simulink model "my_foc_TI"  (R2021b)
settings: Solver=ode23t  StartTime=0.0  StopTime=1  FixedStep=0.0000001  RelTol=1e-7  EnableMultiTasking=on
InitFcn:
  | Ld=5.25e-3;
  | Lq=12e-3;
  | R=0.958;
  | f=0.1827;
model workspace (MAT data in the model file):
  f = Simulink.Signal
  f.DataType = 'single'
  f.Dimensions = 1
  f.DimensionsMode = 'auto'
  f.Complexity = 'real'
  f.SampleTime = -1
  f.SamplingMode = 'auto'
  f.InitialValue = '0.1827'
undefined symbols (not defined in the file or in its folder): sigbuilder_block
libraries: slpidlib x7, simulink x3, SignalEditorBlockLib x2, mcbplantlib x1, spsPermanentMagnetSynchronousMachineLib x1, autolibpmsmexterior x1, spspowerguiLib x1
settings Model: Creator=张豪  LastModifiedBy=LingweiWRB
settings SolverCC: AutoInsertRateTranBlk=on

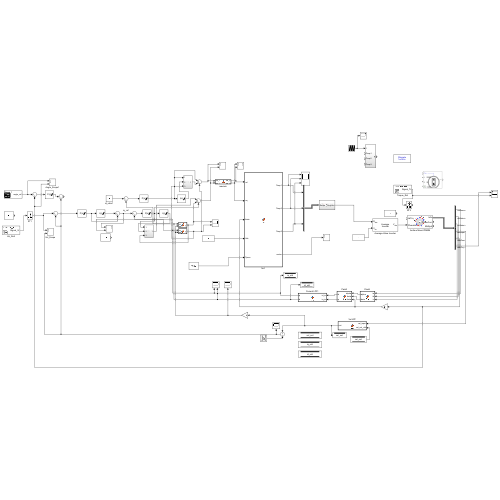
[thumbnail: Simulink's stored preview of the top-level diagram]
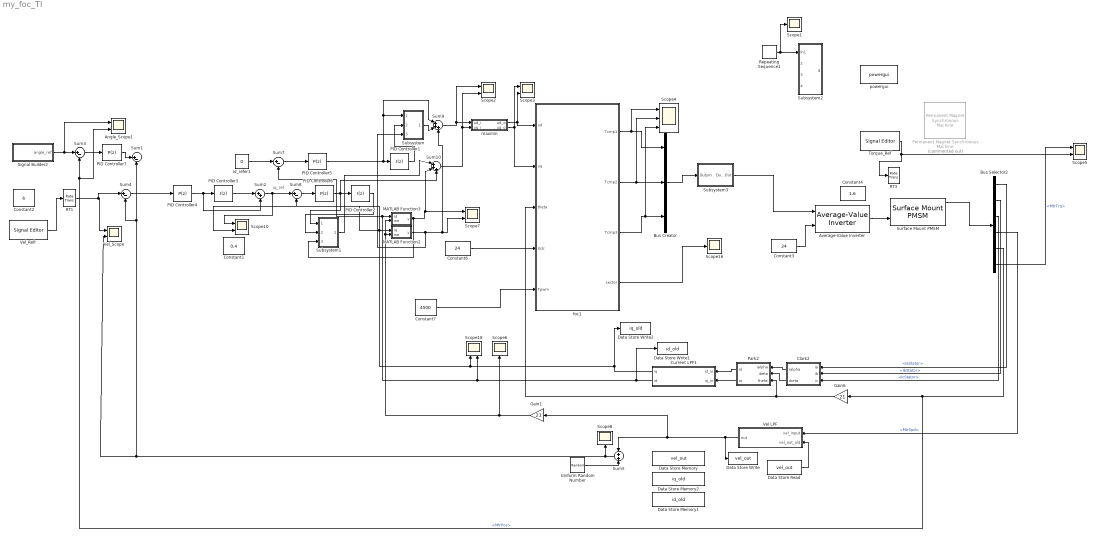
== system my_foc_TI ==
  note: iq_ref
  Angle_Scope1 : Scope  NumInputPorts=2
  Average-Value Inverter : mcbplantlib/Average-Value Inverter
  Bus Creator : BusCreator  Inputs=3
  Bus Selector2 : BusSelector  OutputSignals=IaStator,IbStator,IcStator,MtrSpd,MtrPos,MtrTrq
  Clark2 : MATLAB Function  TreatAsAtomicUnit=on
  Constant1 : Constant  Value=0.4  OutDataTypeStr=single
  Constant2 : Constant  Value=6  OutDataTypeStr=single
  Constant3 : Constant  Value=24
  Constant4 : Constant  Value=1.6
  Constant6 : Constant  Value=24
  Constant7 : Constant  Value=4500  OutDataTypeStr=single
  Current LPF1 : MATLAB Function  TreatAsAtomicUnit=on
  Data Store Memory : DataStoreMemory  DataStoreName=vel_out  ReadBeforeWriteMsg=warning  WriteAfterWriteMsg=warning  WriteAfterReadMsg=warning  ShowAdditionalParam=off  OutDataTypeStr=double
  Data Store Memory1 : DataStoreMemory  DataStoreName=id_old  ReadBeforeWriteMsg=warning  WriteAfterWriteMsg=warning  WriteAfterReadMsg=warning  ShowAdditionalParam=off  OutDataTypeStr=double
  Data Store Memory2 : DataStoreMemory  DataStoreName=iq_old  ReadBeforeWriteMsg=warning  WriteAfterWriteMsg=warning  WriteAfterReadMsg=warning  ShowAdditionalParam=off  OutDataTypeStr=double
  Data Store Read : DataStoreRead  DataStoreName=vel_out  DataStoreElements=vel_out  IndexOptions=Index vector (dialog)  Indices=1  OutputSizes=1
  Data Store Write : DataStoreWrite  DataStoreName=vel_out  DataStoreElements=vel_out  IndexOptions=Index vector (dialog)  Indices=1  OutputSizes=1
  Data Store Write1 : DataStoreWrite  DataStoreName=id_old  DataStoreElements=id_old  IndexOptions=Index vector (dialog)  Indices=1  OutputSizes=1
  Data Store Write2 : DataStoreWrite  DataStoreName=iq_old  DataStoreElements=iq_old  IndexOptions=Index vector (dialog)  Indices=1  OutputSizes=1
  Gain1 : Gain  Gain=21
  Gain6 : Gain  Gain=21
  MATLAB Function2 : MATLAB Function  TreatAsAtomicUnit=on
  MATLAB Function3 : MATLAB Function  TreatAsAtomicUnit=on
  PID Controller1 : slpidlib/PID Controller  Controller=I  Form=Parallel  TimeDomain=Discrete-time  UseExternalTs=off  SampleTime=-1  IntegratorMethod=Forward Euler  FilterMethod=Forward Euler  ControllerParametersSource=internal  P=3.768  I=406.4740  D=0  UseFilter=on  N=100  TunerSelectOption=Transfer Function Based (PID Tuner App)  InitialConditionSource=internal  InitialConditionForIntegrator=0  InitialConditionForFilter=0  DifferentiatorICPrevScaledInput=0  ExternalReset=none  TrackingMode=off  Kt=1  LimitOutput=on  SatLimitsSource=internal  UpperSaturationLimit=36  LowerSaturationLimit=-36  LinearizeAsGain=on  AntiWindupMode=none  Kb=1  POutMin=[]  POutMax=[]  IOutMin=[]  IOutMax=[]  DOutMin=[]  DOutMax=[]  NOutMin=[]  NOutMax=[]  SumOutMin=[]  SumOutMax=[]  SaturationOutMin=[]  SaturationOutMax=[]  PParamMin=[]  PParamMax=[]  IParamMin=[]  IParamMax=[]  DParamMin=[]  DParamMax=[]  NParamMin=[]  NParamMax=[]  KbParamMin=[]  KbParamMax=[]  KtParamMin=[]  KtParamMax=[]  KbOutMin=[]  KbOutMax=[]  KtOutMin=[]  KtOutMax=[]  IntegratorOutMin=[]  IntegratorOutMax=[]  FilterOutMin=[]  FilterOutMax=[]  SumI1OutMin=[]  SumI1OutMax=[]  SumI2OutMin=[]  SumI2OutMax=[]  SumI3OutMin=[]  SumI3OutMax=[]  SumI4OutMin=[]  SumI4OutMax=[]  SumDOutMin=[]  SumDOutMax=[]  DifferentiatorOutMin=[]  DifferentiatorOutMax=[]  FilterDiffOutCoefMin=[]  FilterDiffOutCoefMax=[]  ReciprocalOutMin=[]  ReciprocalOutMax=[]  SumDenOutMin=[]  SumDenOutMax=[]  SumNumOutMin=[]  SumNumOutMax=[]  DivideOutMin=[]  DivideOutMax=[]  UdiffTsProdOutMin=[]  UdiffTsProdOutMax=[]  NTsProdOutMin=[]  NTsProdOutMax=[]  UintegralTsProdOutMin=[]  UintegralTsProdOutMax=[]  UngainTsProdOutMin=[]  UngainTsProdOutMax=[]  IntegratorContinuousStateAttributes=''  IntegratorStateMustResolveToSignalObject=off  IntegratorRTWStateStorageClass=Auto  FilterContinuousStateAttributes=''  FilterStateMustResolveToSignalObject=off  FilterRTWStateStorageClass=Auto  ParallelPVariant=Disabled  IdealPVariant=Disabled  IVariant=InternalParameters  DVariant=Disabled  IntegratorVariant=Discrete  SatVariant=Enabled  AWVariant=Passthrough  PCopyVariant=Disabled  TRVariant=Disabled  FdbkBlocksVariant=Forward  IdealPFdbkVariant=Disabled  SatFdbkVariant=Disabled  DerivativeFilterVariant=Disabled  NVariant=Disabled  NCopyVariant=Disabled_SignalSpec  FilterICVariant=Disabled  IntegratorICVariant=InternalICs  ExternalResetVariant=Disabled  TRSumVariant=Passthrough  SumFdbkVariant=Disabled  SumVariant=Passthrough_I  TsampFilterVariant=InternalTs  TsampNgainVariant=Passthrough  TsampIntegralVariant=Passthrough  ExternalSaturationOutDataTypeStr=Inherit: Same as second input
  PID Controller2 : slpidlib/PID Controller  Controller=I  Form=Parallel  TimeDomain=Discrete-time  UseExternalTs=off  SampleTime=-1  IntegratorMethod=Forward Euler  FilterMethod=Forward Euler  ControllerParametersSource=internal  P=3.768  I=406.4740  D=0  UseFilter=on  N=100  TunerSelectOption=Transfer Function Based (PID Tuner App)  InitialConditionSource=internal  InitialConditionForIntegrator=0  InitialConditionForFilter=0  DifferentiatorICPrevScaledInput=0  ExternalReset=none  TrackingMode=off  Kt=1  LimitOutput=on  SatLimitsSource=internal  UpperSaturationLimit=36  LowerSaturationLimit=-36  LinearizeAsGain=on  AntiWindupMode=none  Kb=1  POutMin=[]  POutMax=[]  IOutMin=[]  IOutMax=[]  DOutMin=[]  DOutMax=[]  NOutMin=[]  NOutMax=[]  SumOutMin=[]  SumOutMax=[]  SaturationOutMin=[]  SaturationOutMax=[]  PParamMin=[]  PParamMax=[]  IParamMin=[]  IParamMax=[]  DParamMin=[]  DParamMax=[]  NParamMin=[]  NParamMax=[]  KbParamMin=[]  KbParamMax=[]  KtParamMin=[]  KtParamMax=[]  KbOutMin=[]  KbOutMax=[]  KtOutMin=[]  KtOutMax=[]  IntegratorOutMin=[]  IntegratorOutMax=[]  FilterOutMin=[]  FilterOutMax=[]  SumI1OutMin=[]  SumI1OutMax=[]  SumI2OutMin=[]  SumI2OutMax=[]  SumI3OutMin=[]  SumI3OutMax=[]  SumI4OutMin=[]  SumI4OutMax=[]  SumDOutMin=[]  SumDOutMax=[]  DifferentiatorOutMin=[]  DifferentiatorOutMax=[]  FilterDiffOutCoefMin=[]  FilterDiffOutCoefMax=[]  ReciprocalOutMin=[]  ReciprocalOutMax=[]  SumDenOutMin=[]  SumDenOutMax=[]  SumNumOutMin=[]  SumNumOutMax=[]  DivideOutMin=[]  DivideOutMax=[]  UdiffTsProdOutMin=[]  UdiffTsProdOutMax=[]  NTsProdOutMin=[]  NTsProdOutMax=[]  UintegralTsProdOutMin=[]  UintegralTsProdOutMax=[]  UngainTsProdOutMin=[]  UngainTsProdOutMax=[]  IntegratorContinuousStateAttributes=''  IntegratorStateMustResolveToSignalObject=off  IntegratorRTWStateStorageClass=Auto  FilterContinuousStateAttributes=''  FilterStateMustResolveToSignalObject=off  FilterRTWStateStorageClass=Auto  ParallelPVariant=Disabled  IdealPVariant=Disabled  IVariant=InternalParameters  DVariant=Disabled  IntegratorVariant=Discrete  SatVariant=Enabled  AWVariant=Passthrough  PCopyVariant=Disabled  TRVariant=Disabled  FdbkBlocksVariant=Forward  IdealPFdbkVariant=Disabled  SatFdbkVariant=Disabled  DerivativeFilterVariant=Disabled  NVariant=Disabled  NCopyVariant=Disabled_SignalSpec  FilterICVariant=Disabled  IntegratorICVariant=InternalICs  ExternalResetVariant=Disabled  TRSumVariant=Passthrough  SumFdbkVariant=Disabled  SumVariant=Passthrough_I  TsampFilterVariant=InternalTs  TsampNgainVariant=Passthrough  TsampIntegralVariant=Passthrough  ExternalSaturationOutDataTypeStr=Inherit: Same as second input
  PID Controller3 : slpidlib/PID Controller  Controller=I  Form=Parallel  TimeDomain=Discrete-time  UseExternalTs=off  SampleTime=-1  IntegratorMethod=Forward Euler  FilterMethod=Forward Euler  ControllerParametersSource=internal  P=3.768  I=14.1129  D=0  UseFilter=on  N=100  TunerSelectOption=Transfer Function Based (PID Tuner App)  InitialConditionSource=internal  InitialConditionForIntegrator=0  InitialConditionForFilter=0  DifferentiatorICPrevScaledInput=0  ExternalReset=none  TrackingMode=off  Kt=1  LimitOutput=on  SatLimitsSource=internal  UpperSaturationLimit=36  LowerSaturationLimit=-36  LinearizeAsGain=on  AntiWindupMode=none  Kb=1  POutMin=[]  POutMax=[]  IOutMin=[]  IOutMax=[]  DOutMin=[]  DOutMax=[]  NOutMin=[]  NOutMax=[]  SumOutMin=[]  SumOutMax=[]  SaturationOutMin=[]  SaturationOutMax=[]  PParamMin=[]  PParamMax=[]  IParamMin=[]  IParamMax=[]  DParamMin=[]  DParamMax=[]  NParamMin=[]  NParamMax=[]  KbParamMin=[]  KbParamMax=[]  KtParamMin=[]  KtParamMax=[]  KbOutMin=[]  KbOutMax=[]  KtOutMin=[]  KtOutMax=[]  IntegratorOutMin=[]  IntegratorOutMax=[]  FilterOutMin=[]  FilterOutMax=[]  SumI1OutMin=[]  SumI1OutMax=[]  SumI2OutMin=[]  SumI2OutMax=[]  SumI3OutMin=[]  SumI3OutMax=[]  SumI4OutMin=[]  SumI4OutMax=[]  SumDOutMin=[]  SumDOutMax=[]  DifferentiatorOutMin=[]  DifferentiatorOutMax=[]  FilterDiffOutCoefMin=[]  FilterDiffOutCoefMax=[]  ReciprocalOutMin=[]  ReciprocalOutMax=[]  SumDenOutMin=[]  SumDenOutMax=[]  SumNumOutMin=[]  SumNumOutMax=[]  DivideOutMin=[]  DivideOutMax=[]  UdiffTsProdOutMin=[]  UdiffTsProdOutMax=[]  NTsProdOutMin=[]  NTsProdOutMax=[]  UintegralTsProdOutMin=[]  UintegralTsProdOutMax=[]  UngainTsProdOutMin=[]  UngainTsProdOutMax=[]  IntegratorContinuousStateAttributes=''  IntegratorStateMustResolveToSignalObject=off  IntegratorRTWStateStorageClass=Auto  FilterContinuousStateAttributes=''  FilterStateMustResolveToSignalObject=off  FilterRTWStateStorageClass=Auto  ParallelPVariant=Disabled  IdealPVariant=Disabled  IVariant=InternalParameters  DVariant=Disabled  IntegratorVariant=Discrete  SatVariant=Enabled  AWVariant=Passthrough  PCopyVariant=Disabled  TRVariant=Disabled  FdbkBlocksVariant=Forward  IdealPFdbkVariant=Disabled  SatFdbkVariant=Disabled  DerivativeFilterVariant=Disabled  NVariant=Disabled  NCopyVariant=Disabled_SignalSpec  FilterICVariant=Disabled  IntegratorICVariant=InternalICs  ExternalResetVariant=Disabled  TRSumVariant=Passthrough  SumFdbkVariant=Disabled  SumVariant=Passthrough_I  TsampFilterVariant=InternalTs  TsampNgainVariant=Passthrough  TsampIntegralVariant=Passthrough  ExternalSaturationOutDataTypeStr=Inherit: Same as second input
  PID Controller4 : slpidlib/PID Controller  Controller=P  Form=Parallel  TimeDomain=Discrete-time  UseExternalTs=off  SampleTime=-1  IntegratorMethod=Forward Euler  FilterMethod=Forward Euler  ControllerParametersSource=internal  P=1.6026  I=1614.8  D=0  UseFilter=on  N=100  TunerSelectOption=Transfer Function Based (PID Tuner App)  InitialConditionSource=internal  InitialConditionForIntegrator=0  InitialConditionForFilter=0  DifferentiatorICPrevScaledInput=0  ExternalReset=none  TrackingMode=off  Kt=1  LimitOutput=on  SatLimitsSource=internal  UpperSaturationLimit=36  LowerSaturationLimit=-36  LinearizeAsGain=on  AntiWindupMode=none  Kb=1  POutMin=[]  POutMax=[]  IOutMin=[]  IOutMax=[]  DOutMin=[]  DOutMax=[]  NOutMin=[]  NOutMax=[]  SumOutMin=[]  SumOutMax=[]  SaturationOutMin=[]  SaturationOutMax=[]  PParamMin=[]  PParamMax=[]  IParamMin=[]  IParamMax=[]  DParamMin=[]  DParamMax=[]  NParamMin=[]  NParamMax=[]  KbParamMin=[]  KbParamMax=[]  KtParamMin=[]  KtParamMax=[]  KbOutMin=[]  KbOutMax=[]  KtOutMin=[]  KtOutMax=[]  IntegratorOutMin=[]  IntegratorOutMax=[]  FilterOutMin=[]  FilterOutMax=[]  SumI1OutMin=[]  SumI1OutMax=[]  SumI2OutMin=[]  SumI2OutMax=[]  SumI3OutMin=[]  SumI3OutMax=[]  SumI4OutMin=[]  SumI4OutMax=[]  SumDOutMin=[]  SumDOutMax=[]  DifferentiatorOutMin=[]  DifferentiatorOutMax=[]  FilterDiffOutCoefMin=[]  FilterDiffOutCoefMax=[]  ReciprocalOutMin=[]  ReciprocalOutMax=[]  SumDenOutMin=[]  SumDenOutMax=[]  SumNumOutMin=[]  SumNumOutMax=[]  DivideOutMin=[]  DivideOutMax=[]  UdiffTsProdOutMin=[]  UdiffTsProdOutMax=[]  NTsProdOutMin=[]  NTsProdOutMax=[]  UintegralTsProdOutMin=[]  UintegralTsProdOutMax=[]  UngainTsProdOutMin=[]  UngainTsProdOutMax=[]  IntegratorContinuousStateAttributes=''  IntegratorStateMustResolveToSignalObject=off  IntegratorRTWStateStorageClass=Auto  FilterContinuousStateAttributes=''  FilterStateMustResolveToSignalObject=off  FilterRTWStateStorageClass=Auto  ParallelPVariant=InternalParameters  IdealPVariant=Disabled  IVariant=Disabled  DVariant=Disabled  IntegratorVariant=Disabled  SatVariant=Enabled  AWVariant=Disabled  PCopyVariant=Disabled  TRVariant=Disabled  FdbkBlocksVariant=Forward  IdealPFdbkVariant=Disabled  SatFdbkVariant=Disabled  DerivativeFilterVariant=Disabled  NVariant=Disabled  NCopyVariant=Disabled_SignalSpec  FilterICVariant=Disabled  IntegratorICVariant=Disabled  ExternalResetVariant=Disabled  TRSumVariant=Passthrough  SumFdbkVariant=Disabled  SumVariant=Passthrough_P  TsampFilterVariant=InternalTs  TsampNgainVariant=Passthrough  TsampIntegralVariant=Disabled_SignalSpec  ExternalSaturationOutDataTypeStr=Inherit: Same as second input
  PID Controller5 : slpidlib/PID Controller  Controller=P  Form=Parallel  TimeDomain=Discrete-time  UseExternalTs=off  SampleTime=-1  IntegratorMethod=Forward Euler  FilterMethod=Forward Euler  ControllerParametersSource=internal  P=0.1384  I=1614.8  D=0  UseFilter=on  N=100  TunerSelectOption=Transfer Function Based (PID Tuner App)  InitialConditionSource=internal  InitialConditionForIntegrator=0  InitialConditionForFilter=0  DifferentiatorICPrevScaledInput=0  ExternalReset=none  TrackingMode=off  Kt=1  LimitOutput=on  SatLimitsSource=internal  UpperSaturationLimit=36  LowerSaturationLimit=-36  LinearizeAsGain=on  AntiWindupMode=none  Kb=1  POutMin=[]  POutMax=[]  IOutMin=[]  IOutMax=[]  DOutMin=[]  DOutMax=[]  NOutMin=[]  NOutMax=[]  SumOutMin=[]  SumOutMax=[]  SaturationOutMin=[]  SaturationOutMax=[]  PParamMin=[]  PParamMax=[]  IParamMin=[]  IParamMax=[]  DParamMin=[]  DParamMax=[]  NParamMin=[]  NParamMax=[]  KbParamMin=[]  KbParamMax=[]  KtParamMin=[]  KtParamMax=[]  KbOutMin=[]  KbOutMax=[]  KtOutMin=[]  KtOutMax=[]  IntegratorOutMin=[]  IntegratorOutMax=[]  FilterOutMin=[]  FilterOutMax=[]  SumI1OutMin=[]  SumI1OutMax=[]  SumI2OutMin=[]  SumI2OutMax=[]  SumI3OutMin=[]  SumI3OutMax=[]  SumI4OutMin=[]  SumI4OutMax=[]  SumDOutMin=[]  SumDOutMax=[]  DifferentiatorOutMin=[]  DifferentiatorOutMax=[]  FilterDiffOutCoefMin=[]  FilterDiffOutCoefMax=[]  ReciprocalOutMin=[]  ReciprocalOutMax=[]  SumDenOutMin=[]  SumDenOutMax=[]  SumNumOutMin=[]  SumNumOutMax=[]  DivideOutMin=[]  DivideOutMax=[]  UdiffTsProdOutMin=[]  UdiffTsProdOutMax=[]  NTsProdOutMin=[]  NTsProdOutMax=[]  UintegralTsProdOutMin=[]  UintegralTsProdOutMax=[]  UngainTsProdOutMin=[]  UngainTsProdOutMax=[]  IntegratorContinuousStateAttributes=''  IntegratorStateMustResolveToSignalObject=off  IntegratorRTWStateStorageClass=Auto  FilterContinuousStateAttributes=''  FilterStateMustResolveToSignalObject=off  FilterRTWStateStorageClass=Auto  ParallelPVariant=InternalParameters  IdealPVariant=Disabled  IVariant=Disabled  DVariant=Disabled  IntegratorVariant=Disabled  SatVariant=Enabled  AWVariant=Disabled  PCopyVariant=Disabled  TRVariant=Disabled  FdbkBlocksVariant=Forward  IdealPFdbkVariant=Disabled  SatFdbkVariant=Disabled  DerivativeFilterVariant=Disabled  NVariant=Disabled  NCopyVariant=Disabled_SignalSpec  FilterICVariant=Disabled  IntegratorICVariant=Disabled  ExternalResetVariant=Disabled  TRSumVariant=Passthrough  SumFdbkVariant=Disabled  SumVariant=Passthrough_P  TsampFilterVariant=InternalTs  TsampNgainVariant=Passthrough  TsampIntegralVariant=Disabled_SignalSpec  ExternalSaturationOutDataTypeStr=Inherit: Same as second input
  PID Controller6 : slpidlib/PID Controller  Controller=P  Form=Parallel  TimeDomain=Discrete-time  UseExternalTs=off  SampleTime=-1  IntegratorMethod=Forward Euler  FilterMethod=Forward Euler  ControllerParametersSource=internal  P=0.1384  I=1614.8  D=0  UseFilter=on  N=100  TunerSelectOption=Transfer Function Based (PID Tuner App)  InitialConditionSource=internal  InitialConditionForIntegrator=0  InitialConditionForFilter=0  DifferentiatorICPrevScaledInput=0  ExternalReset=none  TrackingMode=off  Kt=1  LimitOutput=on  SatLimitsSource=internal  UpperSaturationLimit=36  LowerSaturationLimit=-36  LinearizeAsGain=on  AntiWindupMode=none  Kb=1  POutMin=[]  POutMax=[]  IOutMin=[]  IOutMax=[]  DOutMin=[]  DOutMax=[]  NOutMin=[]  NOutMax=[]  SumOutMin=[]  SumOutMax=[]  SaturationOutMin=[]  SaturationOutMax=[]  PParamMin=[]  PParamMax=[]  IParamMin=[]  IParamMax=[]  DParamMin=[]  DParamMax=[]  NParamMin=[]  NParamMax=[]  KbParamMin=[]  KbParamMax=[]  KtParamMin=[]  KtParamMax=[]  KbOutMin=[]  KbOutMax=[]  KtOutMin=[]  KtOutMax=[]  IntegratorOutMin=[]  IntegratorOutMax=[]  FilterOutMin=[]  FilterOutMax=[]  SumI1OutMin=[]  SumI1OutMax=[]  SumI2OutMin=[]  SumI2OutMax=[]  SumI3OutMin=[]  SumI3OutMax=[]  SumI4OutMin=[]  SumI4OutMax=[]  SumDOutMin=[]  SumDOutMax=[]  DifferentiatorOutMin=[]  DifferentiatorOutMax=[]  FilterDiffOutCoefMin=[]  FilterDiffOutCoefMax=[]  ReciprocalOutMin=[]  ReciprocalOutMax=[]  SumDenOutMin=[]  SumDenOutMax=[]  SumNumOutMin=[]  SumNumOutMax=[]  DivideOutMin=[]  DivideOutMax=[]  UdiffTsProdOutMin=[]  UdiffTsProdOutMax=[]  NTsProdOutMin=[]  NTsProdOutMax=[]  UintegralTsProdOutMin=[]  UintegralTsProdOutMax=[]  UngainTsProdOutMin=[]  UngainTsProdOutMax=[]  IntegratorContinuousStateAttributes=''  IntegratorStateMustResolveToSignalObject=off  IntegratorRTWStateStorageClass=Auto  FilterContinuousStateAttributes=''  FilterStateMustResolveToSignalObject=off  FilterRTWStateStorageClass=Auto  ParallelPVariant=InternalParameters  IdealPVariant=Disabled  IVariant=Disabled  DVariant=Disabled  IntegratorVariant=Disabled  SatVariant=Enabled  AWVariant=Disabled  PCopyVariant=Disabled  TRVariant=Disabled  FdbkBlocksVariant=Forward  IdealPFdbkVariant=Disabled  SatFdbkVariant=Disabled  DerivativeFilterVariant=Disabled  NVariant=Disabled  NCopyVariant=Disabled_SignalSpec  FilterICVariant=Disabled  IntegratorICVariant=Disabled  ExternalResetVariant=Disabled  TRSumVariant=Passthrough  SumFdbkVariant=Disabled  SumVariant=Passthrough_P  TsampFilterVariant=InternalTs  TsampNgainVariant=Passthrough  TsampIntegralVariant=Disabled_SignalSpec  ExternalSaturationOutDataTypeStr=Inherit: Same as second input
  PID Controller7 : slpidlib/PID Controller  Controller=P  Form=Parallel  TimeDomain=Discrete-time  UseExternalTs=off  SampleTime=-1  IntegratorMethod=Forward Euler  FilterMethod=Forward Euler  ControllerParametersSource=internal  P=10  I=1000  D=1  UseFilter=on  N=100  TunerSelectOption=Transfer Function Based (PID Tuner App)  InitialConditionSource=internal  InitialConditionForIntegrator=0  InitialConditionForFilter=0  DifferentiatorICPrevScaledInput=0  ExternalReset=none  TrackingMode=off  Kt=1  LimitOutput=on  SatLimitsSource=internal  UpperSaturationLimit=36  LowerSaturationLimit=-36  LinearizeAsGain=on  AntiWindupMode=none  Kb=1  POutMin=[]  POutMax=[]  IOutMin=[]  IOutMax=[]  DOutMin=[]  DOutMax=[]  NOutMin=[]  NOutMax=[]  SumOutMin=[]  SumOutMax=[]  SaturationOutMin=[]  SaturationOutMax=[]  PParamMin=[]  PParamMax=[]  IParamMin=[]  IParamMax=[]  DParamMin=[]  DParamMax=[]  NParamMin=[]  NParamMax=[]  KbParamMin=[]  KbParamMax=[]  KtParamMin=[]  KtParamMax=[]  KbOutMin=[]  KbOutMax=[]  KtOutMin=[]  KtOutMax=[]  IntegratorOutMin=[]  IntegratorOutMax=[]  FilterOutMin=[]  FilterOutMax=[]  SumI1OutMin=[]  SumI1OutMax=[]  SumI2OutMin=[]  SumI2OutMax=[]  SumI3OutMin=[]  SumI3OutMax=[]  SumI4OutMin=[]  SumI4OutMax=[]  SumDOutMin=[]  SumDOutMax=[]  DifferentiatorOutMin=[]  DifferentiatorOutMax=[]  FilterDiffOutCoefMin=[]  FilterDiffOutCoefMax=[]  ReciprocalOutMin=[]  ReciprocalOutMax=[]  SumDenOutMin=[]  SumDenOutMax=[]  SumNumOutMin=[]  SumNumOutMax=[]  DivideOutMin=[]  DivideOutMax=[]  UdiffTsProdOutMin=[]  UdiffTsProdOutMax=[]  NTsProdOutMin=[]  NTsProdOutMax=[]  UintegralTsProdOutMin=[]  UintegralTsProdOutMax=[]  UngainTsProdOutMin=[]  UngainTsProdOutMax=[]  IntegratorContinuousStateAttributes=''  IntegratorStateMustResolveToSignalObject=off  IntegratorRTWStateStorageClass=Auto  FilterContinuousStateAttributes=''  FilterStateMustResolveToSignalObject=off  FilterRTWStateStorageClass=Auto  ParallelPVariant=InternalParameters  IdealPVariant=Disabled  IVariant=Disabled  DVariant=Disabled  IntegratorVariant=Disabled  SatVariant=Enabled  AWVariant=Disabled  PCopyVariant=Disabled  TRVariant=Disabled  FdbkBlocksVariant=Forward  IdealPFdbkVariant=Disabled  SatFdbkVariant=Disabled  DerivativeFilterVariant=Disabled  NVariant=Disabled  NCopyVariant=Disabled_SignalSpec  FilterICVariant=Disabled  IntegratorICVariant=Disabled  ExternalResetVariant=Disabled  TRSumVariant=Passthrough  SumFdbkVariant=Disabled  SumVariant=Passthrough_P  TsampFilterVariant=InternalTs  TsampNgainVariant=Passthrough  TsampIntegralVariant=Disabled_SignalSpec  ExternalSaturationOutDataTypeStr=Inherit: Same as second input
  Park2 : MATLAB Function  TreatAsAtomicUnit=on
  Permanent Magnet Synchronous Machine : spsPermanentMagnetSynchronousMachineLib/Permanent Magnet Synchronous Machine  Commented=on  NbPhases=3  FluxDistribution=Sinusoidal  RotorType=Round  MechanicalLoad=Torque Tm  PresetModel=No  ShowDetailedParameters=on  MeasurementBus=off  Resistance=0.073  Inductance=8.5e-3  dqInductances=[8.5e-3,8.5e-3]  La=8.65e-05  MachineConstant=Flux linkage established by magnets (V.s)  Flux=0.00941775  VoltageCst=35.872  TorqueCst=0.29666  Flat=120  Mechanical=[0.00120108 3.03448e-06 21]  PolePairs=4  InitialConditions=[0,0, 0,0]  InitialConditions5ph=[0 0 0 0 0 0]  RefAngle=90 degrees behind phase A axis (modified Park)  IterativeDiscreteModel=Trapezoidal non iterative  TsBlock=-1  TsPowergui=0
  RT1 : RateTransition  OutPortSampleTime=0.001
  RT3 : RateTransition  OutPortSampleTime=0.0005
  Repeating Sequence1 : simulink/Sources/Repeating Sequence  rep_seq_t=[0 0.0000125 0.000025]  rep_seq_y=[2250 0 2250]
  Scope{1,6,8,16} (4 alike) : Scope
  Scope{2..3,5,7,10,18} (6 alike) : Scope  NumInputPorts=2
  Scope4 : Scope  NumInputPorts=3
  Signal Builder2 : Subsystem  Tag=STV Subsys  LoadFcn=sigbuilder_block('load');  StartFcn=sigbuilder_block('start');  StopFcn=sigbuilder_block('stop');  ClipboardFcn=sigbuilder_block('clipboard');  mask(Sigbuilder block){tuvar=[0:10]}
      mask help: Simulink:masks:SigbuilderBlock_MD
      mask init:
      | if ~strcmp(get_param(bdroot(gcbh),'SimulationStatus'),'stopped') tuvar = sigbuilder_block('maskInit'); end
      settings: CopyFcn=sigbuilder_block('copy');  DeleteFcn=sigbuilder_block('delete');  ModelCloseFcn=sigbuilder_block('modelClose');  PreSaveFcn=sigbuilder_block('preSave');  PauseFcn=sigbuilder_block('pause');  ContinueFcn=sigbuilder_block('continue');  NameChangeFcn=sigbuilder_block('namechange');  OpenFcn=sigbuilder_block('open',[5.4 36 1141.2 517.8 ]);  CloseFcn=sigbuilder_block('close');
      mask Display: plot(0, 0, 100, 100,[2, 2, 32, 32, 2], [68, 8, 8, 68, 68],[32, 2], [38, 38], [32, 19, 2],[53, 60, 44], [32, 17, 17, 2],[16, 16, 31, 31]);txt = getActiveGroup(gcbh);text(2, 100, txt,'verticalAlignment', 'top');
  Subsystem : Subsystem
  Subsystem1 : Subsystem
  Subsystem2 : Subsystem
  Subsystem3 : Subsystem
  Sum1 : Sum  Inputs=|+-  AccumDataTypeStr=single
  Sum10 : Sum  Inputs=|+++  OutDataTypeStr=single
  Sum2 : Sum  Inputs=|++
  Sum3 : Sum  Inputs=|+-
  Sum4 : Sum  Inputs=|+-  AccumDataTypeStr=single
  Sum5 : Sum
  Sum7 : Sum  Inputs=|+-
  Sum8 : Sum  Inputs=|+-
  Sum9 : Sum  Inputs=|+++  OutDataTypeStr=single
  Surface Mount PMSM : autolibpmsmexterior/Surface Mount PMSM  port_config=Torque  sim_type=Discrete  Ts=0.000025  FilePath=motor_model  P=21  Rs=0.03516  Ldq_=0.0000865  KConstText=Back-emf constant (Ke):  lambda_pm=0.00941775  Ke=35.872  Kt=1.323  mechanical=[0.0012010759, 4.924e-4, 0]  idq0=[0 0]  theta_init=0  omega_init=0  KConst=0.2205  lambda_pm_calc=0.0094177  RefBlkName='autolibpmsmexterior/Surface Mount PMSM'  aMode=5  Ldq="[0.0017      0.0017]"
      settings: SourceProductBaseCode=PW,DR,MT,UV,VE
  Torque_Ref : SignalEditorBlockLib/Signal Editor  FileName=E:\WorkSpace\BLDC_WorkSpace\vel_ref.mat  ActiveScenario=Scenario_tor  ActiveSignal=Signal_Tr  IsBus=off  OutputBusObjectStr=Bus: BusObject  SampleTime=0.000025  OutputAfterFinalValue=Setting to zero  Unit=inherit  PreserveSignalName=on
  Uniform Random Number : UniformRandomNumber  Minimum=-0.4  Maximum=0.4  SampleTime=0.000025
  Vel LPF : MATLAB Function  TreatAsAtomicUnit=on
  Vel_Refr : SignalEditorBlockLib/Signal Editor  FileName=E:\WorkSpace\BLDC_WorkSpace\vel_ref.mat  ActiveScenario=Scenario_Vel  ActiveSignal=Signal_Vr  IsBus=off  OutputBusObjectStr=Bus: BusObject  SampleTime=0.000025  ZeroCross=off  OutputAfterFinalValue=Setting to zero  Unit=inherit  PreserveSignalName=on
  Vel_Scope : Scope  NumInputPorts=2
  foc1 : MATLAB Function  TreatAsAtomicUnit=on
  id_refer1 : Constant  Value=0
  maxmin : MATLAB Function  TreatAsAtomicUnit=on
  powergui : spspowerguiLib/powergui  Priority=1  SimulationMode=Discrete  SampleTime=0.000001  frequency=60  Iterations=50  frequencyindice=0  Pbase=100e6  ErrMax=1e-4  UnitsV=kV  UnitsW=MW  buscounter=0  FunctionMessages=off  echomessages=off  EnableUseOfTLC=off  CurrentSourceSwitches=off  DisableSnubberDevices=off  DisableRonSwitches=off  DisableVfSwitches=off  DisplayEquations=off  AutomaticDiscreteSolvers=off  SolverType=Tustin/Backward Euler (TBE)  Interpol=off  ExternalGateDelay=off  methode=off  Ts=100  x0status=blocks  SPID=on  SwTol=0  HookPort=off  NonlinearTolerance=1e-4  nMaxIteration=100  ContinueOnMaxIteration=off  RestoreLinks=warning  ResistiveCurrentMeasurement=off  Frange=[0:2:500]  Ylog=off  Xlog=on  ShowGrid=off  save=off  variable=ZData  structure=0  ZoomFFT=off  StartTime=0.0  cycles=1  DisplayStyle=1  fundamental=60  FreqAxis=off  MaxFrequency=1000  frequencyindicesteady=1  RmsSteady=1  display=off
  wires:
  Constant7/1 -> foc1/5(Tpwm)
  Constant6/1 -> foc1/4(Udc)
  foc1/4(sector) -> Scope16/1
  Clark2/1(ialpha) -> Park2/1(ialpha)
  Clark2/2(ibeta) -> Park2/2(ibeta)
  Sum7/1 -> PID Controller5/1
  Sum8/1 -> PID Controller6/1
  id_refer1/1 -> Sum7/1
  MATLAB Function3/1(y) -> Subsystem1/3(3), Scope7/1, Sum10/2
  Sum9/1 -> maxmin/1(ud_i), Scope2/1
  Sum10/1 -> maxmin/2(uq_i), Scope2/2
  Gain6/1 -> foc1/3(theta), Park2/3(theta)
  PID Controller5/1 -> Sum9/1, Subsystem/1(In1), PID Controller1/1
  PID Controller6/1 -> Subsystem1/1(In1), Sum10/3, PID Controller2/1
  MATLAB Function2/1(y) -> Subsystem/3(3), Sum9/3, Scope7/2
  Repeating Sequence1/1 -> Scope1/1, Subsystem2/1(In1)
  PID Controller4/1 -> Sum2/2, PID Controller3/1
  PID Controller3/1 -> Sum2/1
  Data Store Read/1 -> Vel LPF/2(vel_out_old)
  PID Controller1/1 -> Subsystem/2(In2)
  Subsystem/1(Out1) -> Sum9/2
  PID Controller2/1 -> Subsystem1/2(In2)
  Subsystem1/1(Out1) -> Sum10/1
  Signal Builder2/1(angle_ref) -> Angle_Scope1/1, Sum3/1
  Sum3/1 -> PID Controller7/1
  RT1/1 -> Sum4/1, Vel_Scope/1
  Vel LPF/1(out) -> Gain1/1, Sum5/1, Data Store Write/1
  Sum5/1 -> Scope8/1, Sum4/2, Sum1/2, Vel_Scope/2
  maxmin/1(ud_o) -> foc1/1(ud), Scope3/2
  maxmin/2(uq_o) -> foc1/2(uq), Scope3/1
  Gain1/1 -> Scope6/1, MATLAB Function3/2(we), MATLAB Function2/2(we)
  Torque_Ref/1 -> RT3/1, Scope5/2
  Current LPF1/2(id) -> Scope18/2, Sum7/2, MATLAB Function3/1(id), Data Store Write1/1
  Vel_Refr/1 -> RT1/1
  Uniform Random Number/1 -> Sum5/2
  Average-Value Inverter/1 -> Surface Mount PMSM/2
  Constant3/1 -> Average-Value Inverter/2
  foc1/1(Tcmp1) -> Scope4/1, Bus Creator/1
  foc1/2(Tcmp2) -> Scope4/2, Bus Creator/2
  foc1/3(Tcmp3) -> Scope4/3, Bus Creator/3
  Bus Creator/1 -> Subsystem3/1(DutyIn)
  Subsystem3/1(DutyOut) -> Average-Value Inverter/1
  Surface Mount PMSM/1 -> Bus Selector2/1
  Bus Selector2/1 -> Clark2/1(ia)  "<IaStator>"
  Bus Selector2/2 -> Clark2/2(ib)  "<IbStator>"
  Bus Selector2/3 -> Clark2/3(ic)  "<IcStator>"
  Bus Selector2/5 -> Angle_Scope1/2, Sum3/2, Gain6/1  "<MtrPos>"
  Bus Selector2/4 -> Vel LPF/1(vel_input)  "<MtrSpd>"
  Park2/1(id) -> Current LPF1/1(id_in)
  Park2/2(iq) -> Current LPF1/2(iq_in)
  Current LPF1/1(iq) -> Scope18/1, Scope10/2, Sum8/2, MATLAB Function2/1(iq), Data Store Write2/1
  Bus Selector2/6 -> Scope5/1  "<MtrTrq>"
  Sum2/1 -> Scope10/1, Sum8/1
  PID Controller7/1 -> Sum1/1
  Sum4/1 -> PID Controller4/1

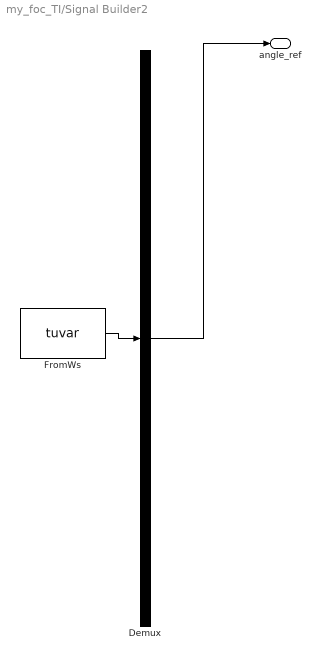
== system my_foc_TI/Signal Builder2 ==
  Demux : Demux  Tag=STV Demux  Outputs=1
      settings: DisplayOption=none
  FromWs : FromWorkspace  Tag=STV FromWs  VariableName=tuvar
      SigBuilderData=|
      | common.afterFinalStr = 'Extrapolate'
      | common.sampleTime = 0
      | dataSet.timeRange = [0 2]
      | dataSet.name = 'Group 1'
      | sbobj.Groups.Name = 'Group 1'
      | sbobj.Groups.Signals.Name = 'angle_ref'
      | sbobj.Groups.Signals.XData = [0 0.1 0.25 0.39 0.4 0.702 0.85 1 1.15 1.3 1.308 1.436 2]
      | sbobj.Groups.Signals.YData = [0.02 0 3.05 3.07 -3.14 -3.04 2.96 3.07 -6.25 -6.32 1.06633846154 1.29083076923 2.28]
      | sbobj.Groups.TimeRange = [0 2]
  angle_ref : Outport  Tag=STV Outport
  wires:
  Demux/1 -> angle_ref/1
  FromWs/1 -> Demux/1

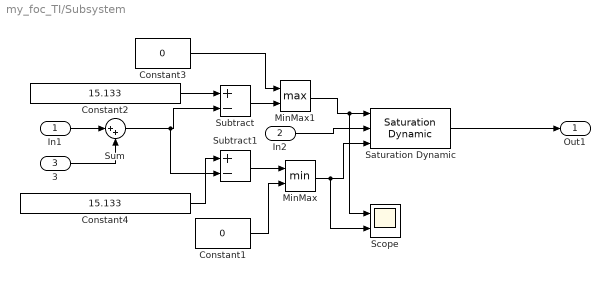
== system my_foc_TI/Subsystem ==
  In1 : Inport
  In2 : Inport  Port=2
  3 : Inport  Port=3
  Constant1 : Constant  Value=0
  Constant2 : Constant  Value=15.133
  Constant3 : Constant  Value=0
  Constant4 : Constant  Value=15.133
  MinMax : MinMax  Inputs=2
  MinMax1 : MinMax  Function=max  Inputs=2
  Saturation Dynamic : simulink/Discontinuities/Saturation Dynamic  OutMin=[]  OutMax=[]  OutDataTypeStr=Inherit: Same as second input  OutDataType=fixdt(1, 16)  OutScaling=2^-10  DoSatur=off
  Scope : Scope  NumInputPorts=2
  Subtract : Sum  Inputs=+-
  Subtract1 : Sum  Inputs=+-
  Sum : Sum  Inputs=|++
  Out1 : Outport
  wires:
  Constant2/1 -> Subtract/1
  Constant3/1 -> MinMax1/1
  In2/1 -> Saturation Dynamic/2
  Subtract/1 -> MinMax1/2
  Saturation Dynamic/1 -> Out1/1
  MinMax1/1 -> Scope/1, Saturation Dynamic/1
  Constant4/1 -> Subtract1/1
  Subtract1/1 -> MinMax/1
  Constant1/1 -> MinMax/2
  MinMax/1 -> Scope/2, Saturation Dynamic/3
  3/1 -> Sum/2
  In1/1 -> Sum/1
  Sum/1 -> Subtract1/2, Subtract/2

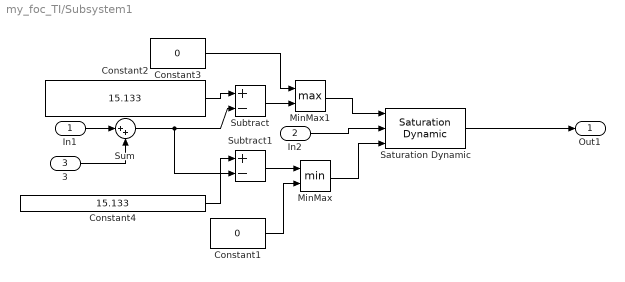
== system my_foc_TI/Subsystem1 ==
  In1 : Inport
  In2 : Inport  Port=2
  3 : Inport  Port=3
  Constant1 : Constant  Value=0
  Constant2 : Constant  Value=15.133
  Constant3 : Constant  Value=0
  Constant4 : Constant  Value=15.133
  MinMax : MinMax  Inputs=2
  MinMax1 : MinMax  Function=max  Inputs=2
  Saturation Dynamic : simulink/Discontinuities/Saturation Dynamic  OutMin=[]  OutMax=[]  OutDataTypeStr=Inherit: Same as second input  OutDataType=fixdt(1, 16)  OutScaling=2^-10  DoSatur=off
  Subtract : Sum  Inputs=+-
  Subtract1 : Sum  Inputs=+-
  Sum : Sum  Inputs=|++
  Out1 : Outport
  wires:
  Constant2/1 -> Subtract/1
  Constant3/1 -> MinMax1/1
  In2/1 -> Saturation Dynamic/2
  Subtract/1 -> MinMax1/2
  Saturation Dynamic/1 -> Out1/1
  MinMax1/1 -> Saturation Dynamic/1
  Constant4/1 -> Subtract1/1
  Subtract1/1 -> MinMax/1
  Constant1/1 -> MinMax/2
  MinMax/1 -> Saturation Dynamic/3
  In1/1 -> Sum/1
  3/1 -> Sum/2
  Sum/1 -> Subtract1/2, Subtract/2

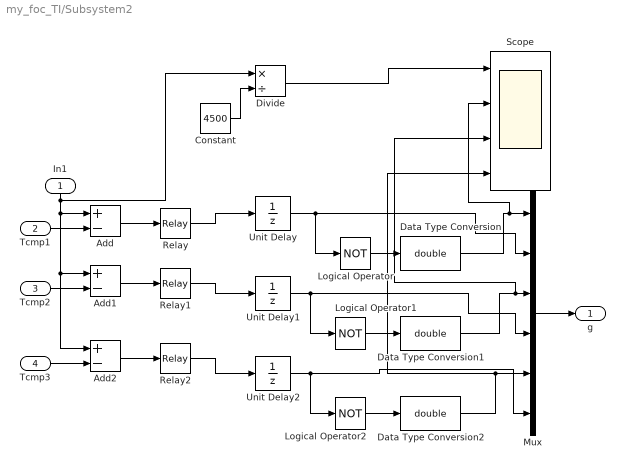
== system my_foc_TI/Subsystem2 ==
  In1 : Inport
  Tcmp1 : Inport  Port=2
  Tcmp2 : Inport  Port=3
  Tcmp3 : Inport  Port=4
  Add : Sum  Inputs=+-
  Add1 : Sum  Inputs=+-
  Add2 : Sum  Inputs=+-
  Constant : Constant  Value=4500
  Data Type Conversion : DataTypeConversion  OutDataTypeStr=double
  Data Type Conversion1 : DataTypeConversion  OutDataTypeStr=double
  Data Type Conversion2 : DataTypeConversion  OutDataTypeStr=double
  Divide : Product  Inputs=*/
  Logical Operator : Logic  Operator=NOT  AllPortsSameDT=off  OutDataTypeStr=boolean
  Logical Operator1 : Logic  Operator=NOT  AllPortsSameDT=off  OutDataTypeStr=boolean
  Logical Operator2 : Logic  Operator=NOT  AllPortsSameDT=off  OutDataTypeStr=boolean
  Mux : Mux  Inputs=6
  Relay : Relay  OffSwitchValue=-eps
  Relay1 : Relay  OffSwitchValue=-eps
  Relay2 : Relay  OffSwitchValue=-eps
  Scope : Scope  NumInputPorts=4
  Unit Delay : UnitDelay  SampleTime=-1  HasFrameUpgradeWarning=on
  Unit Delay1 : UnitDelay  SampleTime=-1  HasFrameUpgradeWarning=on
  Unit Delay2 : UnitDelay  SampleTime=-1  HasFrameUpgradeWarning=on
  g : Outport  VectorParamsAs1DForOutWhenUnconnected=off
  wires:
  Tcmp3/1 -> Add2/2
  Tcmp2/1 -> Add1/2
  Tcmp1/1 -> Add/2
  Relay2/1 -> Unit Delay2/1
  Relay1/1 -> Unit Delay1/1
  Relay/1 -> Unit Delay/1
  Unit Delay2/1 -> Mux/6, Logical Operator2/1
  Unit Delay1/1 -> Mux/4, Logical Operator1/1
  Unit Delay/1 -> Logical Operator/1, Mux/2
  Mux/1 -> g/1
  Logical Operator2/1 -> Data Type Conversion2/1
  Logical Operator1/1 -> Data Type Conversion1/1
  Logical Operator/1 -> Data Type Conversion/1
  Add1/1 -> Relay1/1
  Add2/1 -> Relay2/1
  Add/1 -> Relay/1
  In1/1 -> Divide/1, Add/1, Add2/1, Add1/1
  Constant/1 -> Divide/2
  Divide/1 -> Scope/1
  Data Type Conversion/1 -> Scope/2, Mux/1
  Data Type Conversion1/1 -> Scope/3, Mux/3
  Data Type Conversion2/1 -> Mux/5, Scope/4

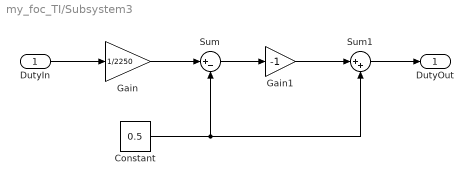
== system my_foc_TI/Subsystem3 ==
  DutyIn : Inport
  Constant : Constant  Value=0.5  SampleTime=-1
  Gain : Gain  Gain=1/2250  ParamDataTypeStr=single
  Gain1 : Gain  Gain=-1
  Sum : Sum  Inputs=|+-
  Sum1 : Sum  Inputs=|++
  DutyOut : Outport
  wires:
  Sum/1 -> Gain1/1
  Constant/1 -> Sum1/2, Sum/2
  DutyIn/1 -> Gain/1
  Gain1/1 -> Sum1/1
  Sum1/1 -> DutyOut/1
  Gain/1 -> Sum/1

== matlab function my_foc_TI/Vel LPF ==
  settings: updateMethod=DISCRETE  sampleTime=0.000025
  data: vel_input input; out output; vel_out data_store_memory; vel_out_old input
function out  = fcn(vel_input, vel_out_old)

out = (1-0.239057223610688)*vel_out_old +0.239057223610688* vel_input;

== matlab function my_foc_TI/maxmin ==
  settings: updateMethod=DISCRETE  sampleTime=0.000025
  data: ud_i input single; f data_store_memory; ud_o output single; uq_i input; uq_o output
function [ud_o, uq_o] = fcn(ud_i, uq_i)

limit = sqrt(ud_i * ud_i + uq_i * uq_i);

if(limit > 15.133)
    ud_o = 15.133 / limit * ud_i;
    uq_o = 15.133 / limit * uq_i;
else
    ud_o = ud_i;
    uq_o = uq_i;
end

end

== matlab function my_foc_TI/Current LPF1 ==
  settings: updateMethod=DISCRETE  sampleTime=0.000025
  data: iq output; id_old data_store_memory; id output; id_in input; iq_in input; iq_old data_store_memory
function [iq,id]  = fcn(id_in, iq_in)
global iq_old;
global id_old;
id = (1-0.38586954)*id_old + 0.38586954* id_in;
iq = (1-0.38586954)*iq_old + 0.38586954* iq_in;
end

== matlab function my_foc_TI/Clark2 ==
  settings: updateMethod=DISCRETE  sampleTime=0.000025
  data: ia input; ialpha output; ib input; ic input; ibeta output
function [ialpha,ibeta] = fcn(ia,ib,ic)
ialpha = ia*2/3-(ib+ic)/3;
ibeta = (ib-ic)*sqrt(3)/3;

== matlab function my_foc_TI/Park2 ==
  settings: updateMethod=DISCRETE  sampleTime=0.000025
  data: ialpha input; ibeta input; theta input; id output; iq output
function [id,iq] = fcn(ialpha,ibeta,theta)
id = ialpha*cos(theta)+ibeta*sin(theta);
iq = -ialpha*sin(theta)+ibeta*cos(theta);

== matlab function my_foc_TI/MATLAB Function2 ==
  settings: updateMethod=DISCRETE  sampleTime=0.000025
  data: iq input; y output; we input; f data_store_memory
function y = fcn(iq,we)

y = -we*iq*0.0000865;

== matlab function my_foc_TI/MATLAB Function3 ==
  settings: updateMethod=DISCRETE  sampleTime=0.000025
  data: id input; we input; f data_store_memory; y output
function y = fcn(id, we)

y = we*(0.00941775+0.0000865*id);

== matlab function my_foc_TI/foc1 ==
  settings: updateMethod=DISCRETE  sampleTime=0.000025
  data: ud input; Tcmp1 output; uq input; theta input; Udc input; Tpwm input; Tcmp2 output; Tcmp3 output; sector output
function [Tcmp1,Tcmp2,Tcmp3,sector] = fcn(ud,uq,theta,Udc,Tpwm)
Valpha = ud*cos(theta) - uq*sin(theta);
Vbeta = ud*sin(theta) + uq*cos(theta);
AAR = Tpwm / 2;
%#codegen

sector = single(0);
Tcmp1 = single(0);
Tcmp2 = single(0);
Tcmp3 = single(0);

%========Parameters statement================

    Vref1 = Vbeta;							                   
    Vref2 = (sqrt(3)*Valpha - Vbeta)/2; 				    
    Vref3 = (-sqrt(3)*Valpha - Vbeta)/2;					
   
 %========Sector calculation=================

  if (Vref1>0)
	   sector = single(1);
  end
  if (Vref2>0)
	   sector = sector+single(2);
  end
  if (Vref3>0)
       sector = sector+single(4);
  end

%======== X Y Z calculation===================

X = sqrt(3)*Vbeta*Tpwm/(Udc*1.15);
Y = Tpwm/(Udc*1.15)*(3/2*Valpha+sqrt(3)/2*Vbeta);
Z = Tpwm/(Udc*1.15)*(-3/2*Valpha+sqrt(3)/2*Vbeta);	         

%==========Duty ratio calculation================
switch (sector)   
    case 1
        T1 = Z; T2 = Y; 
	case 2
        T1 = Y; T2 = -X; 
	case 3
        T1 = -Z; T2 = X; 
	case 4
        T1 = -X; T2 = Z;
	case 5
        T1 = X; T2 = -Y;
    otherwise
        T1 = -Y; T2 = -Z;
end

if T1+T2 > Tpwm
    T1 = T1/(T1+T2);
    T2 = T2/(T1+T2);
else
    T1 = T1;
    T2 = T2;
end

%ccr
ta = (Tpwm-(T1+T2))/4.0;
tb = ta+T1/2;
tc = tb+T2/2;

%%实际代码需要加上
%%ta = AAR -ta;
%%tb = AAR -tb;
%%tc = AAR -tc;

%==========Duty ratio calculation================
switch (sector)
    case 1 
        Tcmp1=tb;
        Tcmp2=ta;
        Tcmp3=tc; 
        
    case 2 
        Tcmp1=ta;
        Tcmp2=tc;
        Tcmp3=tb; 
       
    case 3 
        Tcmp1=ta;
        Tcmp2=tb;
        Tcmp3=tc; 
        
    case 4 
        Tcmp1=tc;
        Tcmp2=tb;
        Tcmp3=ta;
        
    case 5 
        Tcmp1=tc;
        Tcmp2=ta;
        Tcmp3=tb;
        
   case 6
       Tcmp1=tb;
       Tcmp2=tc;
       Tcmp3=ta;
end
end
